simulink model "path_pure_pursuit"  (R2020b)
settings: Solver=VariableStepAuto  StartTime=0.0  StopTime=30.0  RelTol=1e-3
values from neighbouring files (symbols this model uses):
  path = path(1: x(1)-1,:)    [Q_learning_p.m]    (also in path_planner.m = path(1: x(1) - 1,:))
libraries: mobileRoboticsLib x3, robotalgslib x1
settings Model: Creator=Roozbeh  LastModifiedBy=Roozbeh

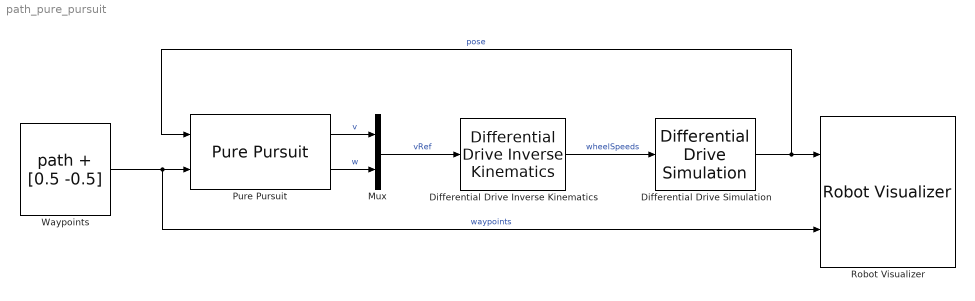
== system path_pure_pursuit ==
  Differential Drive Inverse Kinematics : mobileRoboticsLib/Kinematic Models/Differential Drive/Differential Drive Inverse Kinematics  wheelRadius=0.1  wheelBase=0.5
      settings: SourceProductName=Mobile Robotics Simulation Library
  Differential Drive Simulation : mobileRoboticsLib/Kinematic Models/Differential Drive/Differential Drive Simulation  wheelRadius=0.1  wheelBase=0.5  initX=8  initY=8  initAngle=0  Ts=0.05
      settings: SourceProductName=Mobile Robotics Simulation Library
  Mux : Mux  Inputs=2
  Pure Pursuit : robotalgslib/Pure Pursuit  DesiredLinearVelocity=2  MaxAngularVelocity=1.5  LookaheadDistance=1  TargetDirPort=off  SimulateUsing=Interpreted execution
  Robot Visualizer : mobileRoboticsLib/Environments/Robot Visualizer  Priority=99  robotRadius=0  mapName=mapRooz  showTrajectory=on  hasWaypoints=on  hasLidar=off  sensorOffset=[ 0 0 ]  scanAngles=0  hasObjDetector=off  objDetectorOffset=[ 0, 0 ]  objDetectorAngle=0  objDetectorFOV=0  objDetectorMaxRange=0  objectColors=0  objectMarkers=s
      settings: SourceProductName=Ground Vehicles Library
  Waypoints : Constant  Value=path + [0.5 -0.5]
  wires:
  Pure Pursuit/1 -> Mux/1  "v"
  Differential Drive Inverse Kinematics/1 -> Differential Drive Simulation/1  "wheelSpeeds"
  Mux/1 -> Differential Drive Inverse Kinematics/1  "vRef"
  Differential Drive Simulation/1 -> Pure Pursuit/1, Robot Visualizer/1  "pose"
  Pure Pursuit/2 -> Mux/2  "w"
  Waypoints/1 -> Robot Visualizer/2, Pure Pursuit/2  "waypoints"
